simulink model "Comau_robot_sim_IK_3dof"  (R2024b)
settings: Solver=FixedStepAuto  StartTime=0.0  StopTime=inf  FixedStep=Ts  RelTol=1e-3
model workspace (MATLAB code in the model file):
  other statements: smiDataRobot.RigidTransform(16).translation = [0.0 0.0 0.0];; smiDataRobot.RigidTransform(16).angle = 0.0;; smiDataRobot.RigidTransform(16).axis = [0.0 0.0 0.0];; smiDataRobot.RigidTransform(16).ID = "";; smiDataRobot.RigidTransform(1).translation = [0 331 0];  % mm; smiDataRobot.RigidTransform(1).angle = 0;  % rad; smiDataRobot.RigidTransform(1).axis = [0 0 0];; smiDataRobot.RigidTransform(1).ID = "AssemblyGround[SMART-5 NJ-110-3.0 (3D-STEP).STEP-1:SMART-5 NJ-110-3.0_p02.STEP-1]";; smiDataRobot.RigidTransform(2).translation = [-450 2240 0];  % mm; smiDataRobot.RigidTransform(2).angle = 0;  % rad; smiDataRobot.RigidTransform(2).axis = [0 0 0];; smiDataRobot.RigidTransform(2).ID = "AssemblyGround[SMART-5 NJ-110-3.0 (3D-STEP).STEP-1:SMART-5 NJ-110-3.0_p05.STEP-1]"; ... (+161)
undefined symbols (not defined in the file): L2, L3, L4, M, SList, smiDataRobot, thetaList0, X, Y, Z
libraries: sm_lib x85, nesl_utility x31, slrealtimeutilitieslib x1, slrealtimeiplib x1, aerolibanimutils x1
(part 5 of 5)

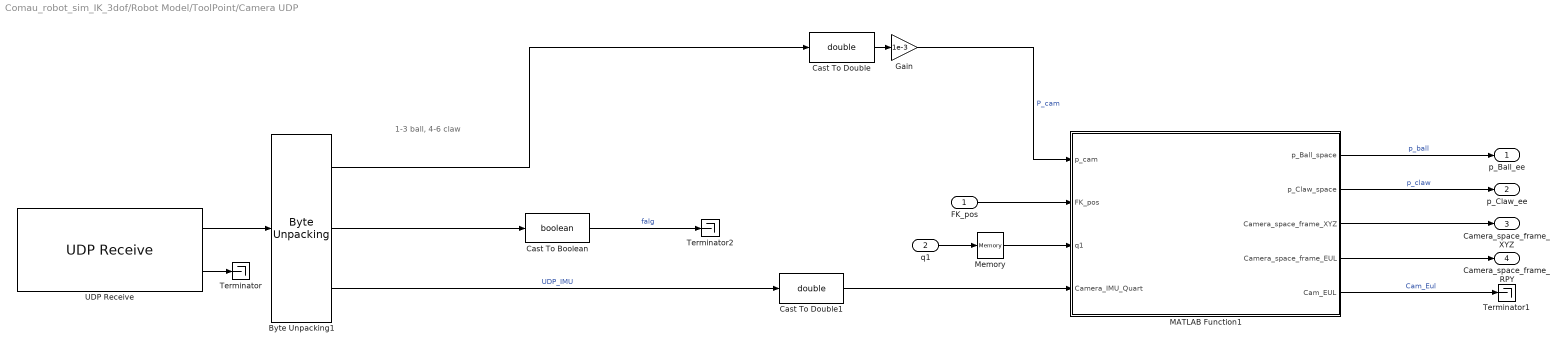
== system Comau_robot_sim_IK_3dof/Robot Model/ToolPoint/Camera UDP ==
  note: 1-3 ball, 4-6 claw
  FK_pos : Inport
  q1 : Inport  Port=2
  Byte Unpacking1 : slrealtimeutilitieslib/Byte Unpacking  MaskUnpackedDataTypes={'int16', 'uint8', 'single'}  MaskUnpackedDataSizes={[6], [1], [4]}  MaskAlignment=1
  Cast To Boolean : DataTypeConversion  OutDataTypeStr=boolean  SaturateOnIntegerOverflow=off  RndMeth=Floor
  Cast To Double : DataTypeConversion  OutDataTypeStr=double  SaturateOnIntegerOverflow=off  RndMeth=Floor
  Cast To Double1 : DataTypeConversion  OutDataTypeStr=double  SaturateOnIntegerOverflow=off  RndMeth=Floor
  Gain : Gain  Gain=1e-3
  MATLAB Function1 : MATLAB Function  TreatAsAtomicUnit=on
  Memory : Memory
  Terminator : Terminator
  Terminator1 : Terminator
  Terminator2 : Terminator
  UDP Receive : slrealtimeiplib/UDP Receive  useHostTargetConn=on  ipAddress=192.168.5.80  localPort=5008  rcvWidth=29  rcvFmAny=on  fmAddress='10.10.10.10'  sampleTime=Ts  enableMessage=off  maxPackets=1
  p_Ball_ee : Outport
  p_Claw_ee : Outport  Port=2
  Camera_space_frame_XYZ : Outport  Port=3
  Camera_space_frame_RPY : Outport  Port=4
  wires:
  Byte Unpacking1/1 -> Cast To Double/1
  Cast To Boolean/1 -> Terminator2/1  "falg"
  UDP Receive/1 -> Byte Unpacking1/1
  UDP Receive/2 -> Terminator/1
  Byte Unpacking1/2 -> Cast To Boolean/1
  Byte Unpacking1/3 -> Cast To Double1/1  "UDP_IMU"
  Gain/1 -> MATLAB Function1/1(p_cam)  "P_cam"
  MATLAB Function1/1(p_Ball_space) -> p_Ball_ee/1  "p_ball"
  MATLAB Function1/2(p_Claw_space) -> p_Claw_ee/1  "p_claw"
  Cast To Double/1 -> Gain/1
  FK_pos/1 -> MATLAB Function1/2(FK_pos)
  MATLAB Function1/3(Camera_space_frame_XYZ) -> Camera_space_frame_XYZ/1
  Cast To Double1/1 -> MATLAB Function1/4(Camera_IMU_Quart)
  MATLAB Function1/4(Camera_space_frame_EUL) -> Camera_space_frame_RPY/1
  q1/1 -> Memory/1
  Memory/1 -> MATLAB Function1/3(q1)
  MATLAB Function1/5(Cam_EUL) -> Terminator1/1  "Cam_Eul"

== matlab function Comau_robot_sim_IK_3dof/TrajectoryGen ==
  settings: updateMethod=DISCRETE
  data: points_x input; points_y input; points_z input; p output size=[1 3]; t input; t_points input; new_command input; traj_method input; p_vel output size=[1 3]; v_max input; traj_running output boolean size=1
function [p, p_vel, traj_running] = TrajectoryGen(points_x, points_y, points_z, t, t_points, new_command, traj_method, v_max)
%#codegen

p = zeros(1, 3);
p_vel = zeros(1, 3);

% Persistent variables for timing and command tracking, and to hold new parameters:
persistent abs_tf base_t last_command 
persistent new_points_x new_points_y new_points_z new_t_points

if isempty(abs_tf)
    base_t = 0;
    abs_tf = 0;
end
if isempty(last_command)
    last_command = 0;
end

% Initialize captured parameters if empty:
if isempty(new_points_x)
    new_points_x = points_x;
end
if isempty(new_points_y)
    new_points_y = points_y;
end
if isempty(new_points_z)
    new_points_z = points_z;
end
if isempty(new_t_points)
    new_t_points = t_points;
end

%Detect a new trajectory command:
if new_command ~= last_command
    %Capture the current time as the start:
    base_t = t;
    
    %Capture the new parameters so they remain consistent:
    new_points_x = points_x;
    new_points_y = points_y;
    new_points_z = points_z;
    
    %Calculate the trajectory duration T based on Vmax.
    %Ensure Vmax is not too small and set a minimum time:
    T_min = 1e-6;
    v_max = max(v_max, T_min);
    
    %For a two-point trajectory, use the difference between the first two points.
    T_x = abs(new_points_x(2) - new_points_x(1)) / v_max;
    T_y = abs(new_points_y(2) - new_points_y(1)) / v_max;
    T_z = abs(new_points_z(2) - new_points_z(1)) / v_max;
    
    %Choose the maximum time required among all three axes:
    T = max([T_x, T_y, T_z, T_min]);
    
    %Set the absolute finish time based on the computed duration:
    abs_tf = T + t;
    
    %store T in new_t_points if needed
    new_t_points = T;  
    
    %Update the command counter:
    last_command = new_command;
end

%Compute local time variables:
local_t = t - base_t;
local_tf = abs_tf - base_t;



%Clamp local_t so it doesn't exceed the final time:
%if traj_method ~= 3
%    if local_t > local_tf
%        local_t = local_tf;
%    end
%end

%Compute the trajectory:
if abs_tf == 0 || v_max == 0 % Stay in current position if Trajectory not initialized OR v_max input = 0
    x_pos = new_points_x(1);
    y_pos = new_points_y(1);
    z_pos = new_points_z(1);
    
    x_vel = 0;
    y_vel = 0;
    z_vel = 0;
else
    if traj_method == 1
        [x_pos, x_vel, ~] = cubicTrajectoryPlanner(local_t, local_tf, new_points_x(1), new_points_x(2), 0, 0);
        [y_pos, y_vel, ~] = cubicTrajectoryPlanner(local_t, local_tf, new_points_y(1), new_points_y(2), 0, 0);
        [z_pos, z_vel, ~] = cubicTrajectoryPlanner(local_t, local_tf, new_points_z(1), new_points_z(2), 0, 0);
        
        %VMax
        %[x_pos, x_vel, ~] = cubicTrajectoryPlanner_Vmax(local_t, v_max, new_points_x(1), new_points_x(2), 0, 0);
        %[y_pos, y_vel, ~] = cubicTrajectoryPlanner_Vmax(local_t, v_max, new_points_y(1), new_points_y(2), 0, 0);
        %[z_pos, z_vel, ~] = cubicTrajectoryPlanner_Vmax(local_t, v_max, new_points_z(1), new_points_z(2), 0, 0);
    elseif traj_method == 2
        %Quintic [pos, vel, acc] = quinticTrajectoryPlanner(t, T, P0, Pf, V0, Vf, A0, Af)
        [x_pos, x_vel, ~] = quinticTrajectoryPlanner(local_t, local_tf, new_points_x(1), new_points_x(2), 0, 0, 0, 0);
        [y_pos, y_vel, ~] = quinticTrajectoryPlanner(local_t, local_tf, new_points_y(1), new_points_y(2), 0, 0, 0, 0);
        [z_pos, z_vel, ~] = quinticTrajectoryPlanner(local_t, local_tf, new_points_z(1), new_points_z(2), 0, 0, 0, 0);
        
        %VMax
        %[x_pos, x_vel, ~] = quinticTrajectoryPlanner_Vmax(local_t, v_max, new_points_x(1), new_points_x(2), 0, 0, 0, 0);
        %[y_pos, y_vel, ~] = quinticTrajectoryPlanner_Vmax(local_t, v_max, new_points_y(1), new_points_y(2), 0, 0, 0, 0);
        %[z_pos, z_vel, ~] = quinticTrajectoryPlanner_Vmax(local_t, v_max, new_points_z(1), new_points_z(2), 0, 0, 0, 0);
    elseif traj_method == 3
        method = 'quintic';
        %Multi point online trajectory planner here
        %[x_pos, x_vel, ~, ~] = multipointTrajectorySplineAuto(local_t, new_points_x, v_max, method);
        %[y_pos, y_vel, ~, ~] = multipointTrajectorySplineAuto(local_t, new_points_y, v_max, method);
        %[z_pos, z_vel, ~, ~] = multipointTrajectorySplineAuto(local_t, new_points_z, v_max, method);

        x_pos = new_points_x(1);
        y_pos = new_points_y(1);
        z_pos = new_points_z(1);
        
        x_vel = 0;
        y_vel = 0;
        z_vel = 0;
    else %Defualt cubic
        [x_pos, x_vel, ~] = cubicTrajectoryPlanner(local_t, local_tf, new_points_x(1), new_points_x(2), 0, 0);
        [y_pos, y_vel, ~] = cubicTrajectoryPlanner(local_t, local_tf, new_points_y(1), new_points_y(2), 0, 0);
        [z_pos, z_vel, ~] = cubicTrajectoryPlanner(local_t, local_tf, new_points_z(1), new_points_z(2), 0, 0);
    end
end


p(1) = x_pos;
p(2) = y_pos;
p(3) = z_pos;

p_vel(1) = x_vel;
p_vel(2) = y_vel;
p_vel(3) = z_vel;

traj_running = (t <= abs_tf + 0.1); %Trajectory complete flag with 0.1 second buffer

traj_running = logical(traj_running);
end

== matlab function Comau_robot_sim_IK_3dof/Robot Model/ToolPoint/Camera UDP/MATLAB Function1 ==
  data: p_Ball_space output; p_Claw_space output; p_cam input; Camera_space_frame_XYZ output; FK_pos input; q1 input; Camera_IMU_Quart input; Camera_space_frame_EUL output; Cam_EUL output
function [p_Ball_space, p_Claw_space, Camera_space_frame_XYZ, Camera_space_frame_EUL, Cam_EUL] = transformFrame(p_cam, FK_pos, q1, Camera_IMU_Quart)

p_Ball_camera = p_cam(1:3);
p_Claw_camera = p_cam(4:6);

% Reorder quaternion from [x; y; z; w] to MATLAB's expected [w, x, y, z]
temp = Camera_IMU_Quart;
q = [temp(4), temp(1), temp(2), temp(3)];
% Convert quaternion to rotation matrix (using MATLAB's Aerospace Toolbox convention)
Cam_EUL = quat2eul(q);
Cam_EUL = rad2deg(Cam_EUL);
R_cam = quat2rotm(q);

% Known translation (offset) from the end effector (EE) to the camera.
t_ee_c = [-0.10; 0; -0.50];
% Combine the IMU rotation with the fixed offset.
T_ee_c = [R_cam, t_ee_c; 0 0 0 1];


% FK_pos end effector position in cartesian space
R_s_ee = rotz(-q1);
T_s_ee = [R_s_ee, FK_pos; 0 0 0 1];


T_s_c = T_s_ee * T_ee_c;

Camera_space_frame_XYZ = T_s_c(1:3,4);
Camera_space_frame_R = T_s_c(1:3,1:3);
Camera_space_frame_EUL = rotm2eul(Camera_space_frame_R, 'XYZ');


R_offset = roty(-pi) * rotz(-pi/2);
T_offset = [R_offset, zeros(3,1); 0 0 0 1];


p_Ball_hom = T_offset * [p_Ball_camera; 1];
p_Claw_hom = T_offset * [p_Claw_camera; 1];

% Transform to the base frame
p_Ball_trans = T_s_c * p_Ball_hom;
p_Claw_trans = T_s_c * p_Claw_hom;
p_Ball_space = p_Ball_trans(1:3);
p_Claw_space = p_Claw_trans(1:3);


% Use persistent variables to store the last valid positions.
persistent p_Ball_space_persistent p_Claw_space_persistent;
if isempty(p_Ball_space_persistent)
    p_Ball_space_persistent = p_Ball_space;
end
if isempty(p_Claw_space_persistent)
    p_Claw_space_persistent = p_Claw_space;
end


bBallInFrame = true;
bClawInFrame = true;
for i = 1:3
    if (abs(p_Ball_camera(i)) >= 20.0) || (abs(p_Ball_camera(i)) <= 0.001)
        bBallInFrame = false;
    end
    if (abs(p_Claw_camera(i)) >= 20.0) || (abs(p_Claw_camera(i)) <= 0.001)
        bClawInFrame = false;
    end
end

% If in frame, update the persistent variable
if bBallInFrame
    p_Ball_space_persistent = p_Ball_space;
else
    p_Ball_space = p_Ball_space_persistent;
end

if bClawInFrame
    p_Claw_space_persistent = p_Claw_space;
else
    p_Claw_space = p_Claw_space_persistent;
end

end

%% 
function R = roty(theta)
R = [ cos(theta)  0 sin(theta);
      0           1 0;
     -sin(theta)  0 cos(theta)];
end

function R = rotz(theta)
R = [cos(theta) -sin(theta) 0;
     sin(theta)  cos(theta) 0;
     0           0          1];
end

== stateflow chart Comau_robot_sim_IK_3dof/Chart ==
  state Go_home
    entry:
    X_home = 2.62;
    Y_home = 0;
    Z_home = 2.24;
    Traj_points_XYZ = [FK_Pos(1), X_home, FK_Pos(2), Y_home, FK_Pos(3), Z_home];
    Traj_method = 2;
    v_max = 0.1;
    new_command = new_command + 1;
  state Stay_in_current_position
    entry:
    % Set the values for the variables
    Traj_points_XYZ = [FK_Pos(1), FK_Pos(1), FK_Pos(2), FK_Pos(2), FK_Pos(3), FK_Pos(3)];
    Traj_method = 1;
    v_max = 0;
    new_command = new_command + 1;
  state Move_to_above_platform
    %Move above platform to initiate hooking procedure
    %Revieve in testing later if this stage is necessery or can be optimized
    entry:
    X_Platform = 3.14;
    Y_Platform = 0.4;
    Z_Platform = 2.0;
    Traj_points_XYZ = [FK_Pos(1), X_Platform, FK_Pos(2), Y_Platform, FK_Pos(3), Z_Platform];
    Traj_method = 2;
    v_max = 0.1;
    new_command = new_command + 1;
  state Hook_Ball
    state Move_Close_To_Ball
      entry:
      X_Offset = -0.24;
      Y_Offset = -0.24;
      Z_Offset = -0.07;
      Target_Pos_X = Ball_Pos(1) + X_Offset;
      Target_Pos_Y = Ball_Pos(2) + Y_Offset;
      Target_Pos_Z = Ball_Pos(3) +  Winch_length; %Z_Offset + Claw_Pos(3);
      Traj_points_XYZ = [FK_Pos(1), Target_Pos_X, FK_Pos(2), Target_Pos_Y, FK_Pos(3), Target_Pos_Z];
      Traj_method = 2;
      v_max = 0.1;
      new_command = new_command + 1;
      during:
      if ~traj_running
      Sub_stage_switch = 2;
      else
      Sub_stage_switch = 1;
      end
    state Ball_In_Frame
      if all(abs(Ball_Pos) < 20)
      Sub_stage_switch = 1;
      else
      Sub_stage_switch = 0;
      v_max = 0;
      end
    state Move_in_to_ball
      entry:
      Traj_points_XYZ = [FK_Pos(1), Ball_Pos(1), FK_Pos(2), Ball_Pos(2), FK_Pos(3), Ball_Pos(3)+Winch_length ];
      Traj_method = 2;
      v_max = 0.02;
      new_command = new_command + 1;
      during:
      if ~traj_running
      Sub_stage_switch = 3;
      else
      Sub_stage_switch = 2;
      end
    state Lift_Up
      entry:
      Z_Up = FK_Pos(3) + 0.20;
      Traj_points_XYZ = [FK_Pos(1), FK_Pos(1), FK_Pos(2), FK_Pos(2), FK_Pos(3), Z_Up ];
      Traj_method = 2;
      v_max = 0.05;
      new_command = new_command + 1;
    (default) -> Ball_In_Frame
    Ball_In_Frame -> Move_Close_To_Ball : [Sub_stage_switch == 1]
    Move_Close_To_Ball -> Move_in_to_ball : [Sub_stage_switch == 2]
    Move_in_to_ball -> Lift_Up : [Sub_stage_switch == 3]
  (default) -> Stay_in_current_position
  Hook_Ball -> Go_home [order 3] : [Switch == 1]
  Stay_in_current_position -> Go_home [order 1] : [Switch == 1]
  Go_home -> Stay_in_current_position [order 1] : [Switch == 0]
  Hook_Ball -> Stay_in_current_position [order 2] : [Switch == 0]
  Move_to_above_platform -> Stay_in_current_position [order 1] : [Switch == 0]
  Stay_in_current_position -> Move_to_above_platform [order 2] : [Switch == 2]
  Move_to_above_platform -> Go_home [order 2] : [Switch == 1]
  Go_home -> Move_to_above_platform [order 2] : [Switch == 2]
  Move_to_above_platform -> Hook_Ball [order 3] : [Switch == 3]
  Hook_Ball -> Move_to_above_platform [order 1] : [Switch==2]
  data: Switch input; Traj_points_XYZ output; new_command output =0; Traj_method output; v_max output =0; FK_Pos input; Claw_Pos input; Z_home local; X_home local; Y_home local; X_Platform local; Z_Platform local; Y_Platform local; Ball_Pos input; Winch_length input; Z_Offset local; X_Offset local; Target_Pos_Y local; Target_Pos_X local; Target_Pos_Z local; Y_Offset local; Sub_stage_switch local; traj_running input; Z_Up local

== matlab function Comau_robot_sim_IK_3dof/MATLAB Function ==
  data: thetalist input; Cartesian_position output; M input; SList input; T output
function [Cartesian_position, T]  = FK_cartPos(thetalist, M, SList)

%Compute end effector frame from Forward kinematics to measure end effector
%position
T = FKinSpace(M,SList,thetalist);

cartPos = [T(1:3,4)];

Cartesian_position = cartPos;

== matlab function Comau_robot_sim_IK_3dof/inverseKinematics ==
  data: p input; thetaList output size=[5, 1]; p_vel input; thetaList0 input; M input; SList input; thetaListDot output size=[5, 1]; success output size=1
function [thetaList, thetaListDot, success] = inverseKinematics( ...
    p, p_vel, thetaList0, M, SList)


T = [1 0 0 p(1);
     0 1 0 p(2);
     0 0 1 p(3);
     0 0 0 1];

[thetaOut, successOut] = IKinSpace(SList, M, T, thetaList0, 0.00001, 0.0000001);


% Assign them to the pre-allocated outputs
thetaList    = thetaOut;
success      = successOut;

%Exploiting linear relationship between q3 and q2 to obtain actual angle of
%of actuated joint
% q3_closure = thetaList(3) - thetaList(2);
% thetaList_closure= [thetaList(1); thetaList(2); q3_closure; thetaList(4); thetaList(5)];


Js = JacobianSpace(SList,thetaList);

%pseudo inverse jacobian
Js_pinv = pinv(Js);
xyzDot = [0;
         0;
         0;
         p_vel(1);
         p_vel(2);
         p_vel(3)
         ];

thetaListDot = Js_pinv*xyzDot;

end
